simulink model "FOC_xeConCauTruc_discrete_251130_DNQ"  (R2024b)
settings: Solver=ode1  StartTime=0.0  StopTime=110  FixedStep=Tsample  MaxStep=1e-3  RelTol=1e-6  EnableMultiTasking=on
values from neighbouring files (symbols this model uses):
  ki1 = kp1/Ti1    (= 1470.9983644)    [parameters.m]    (also in thongso.m = 740.192826747)
  ki2 = kp2/Ti2    (= 348.309892151)    [parameters.m]    (also in thongso.m = 697.25500171)
  kp1 = Ti1/(k*5*(1/4000))    (= 14.8818990391)    [parameters.m]    (also in thongso.m = 10.2896717027)
  kp2 = 2*eta*0.0676/(KT*T0w)    (= 3.04771155633)    [parameters.m]    (also in thongso.m = 4.88078501197)
  Llr = 0.009662862    [parameters.m]    (also in thongso.m = 0.005238655)
  Lls = 0.009662862    [parameters.m]    (also in thongso.m = 0.005238655)
  Lm = 0.1213    [parameters.m]    (also in thongso.m = 0.141018834)
  p = 4    [parameters.m]    (also in thongso.m = 2)
  P = 8    [parameters.m]    (also in thongso.m = 4)
  Rr = 0.97664535    [parameters.m]    (also in thongso.m = 0.380952381)
  Rs = 1.000830856    [parameters.m]    (also in thongso.m = 0.386041637)
  Tr = Lr/Rr    (= 0.134088592138)    [parameters.m]    (also in thongso.m = 0.383925908577)
  Ts = Ls/Rs    (= 0.130848781505)    [parameters.m]    (also in thongso.m = 0.378864544604)
  Tsample = 1e-5    (= 1e-05)    [parameters.m]    (also in thongso.m)
  Vdc = 900    [parameters.m]    (also in thongso.m = 510)
undefined symbols (not defined in the file or in its folder): DiscIntNeverNeededParam, dspblkCoreblockFVToolHelper, gcbh
libraries: powerlib_extras x5, slpidlib x3, spsUniversalBridgeLib x1, spsAsynchronousMachineSIUnitsLib x1, simulink x1, spsVoltageMeasurementLib x1, spsDCVoltageSourceLib x1, sps_lib x1, SignalEditorBlockLib x1
settings Model: Creator=Dell  LastModifiedBy=Admin
settings SolverCC: AlgebraicLoopSolver=TrustRegion
settings DataIOCC: LimitDataPoints=on  SaveFormat=Array  SignalLoggingSaveFormat=ModelDataLogs  ReturnWorkspaceOutputs=off
settings OptimizationCC: ExpressionDepthLimit=2147483647  LifeSpan=inf
settings DebuggingCC: UnderspecifiedInitializationDetection=Classic  MergeDetectMultiDrivingBlocksExec=none  SolverPrmCheckMsg=warning  FcnCallInpInsideContextMsg=warning  UnconnectedInputMsg=warning  UnconnectedOutputMsg=warning  UnconnectedLineMsg=warning  StateNameClashWarn=warning  SFUnexpectedBacktrackingDiag=warning  SFNoUnconditionalDefaultTransitionDiag=warning  ArithmeticOperatorsInVariantConditions=warning
settings HardwareCC: ProdBitPerPointer=32  ProdBitPerSizeT=32  ProdBitPerPtrDiffT=32  ProdLargestAtomicFloat=None  ProdIntDivRoundTo=Undefined  ProdEndianess=Unspecified  ProdWordSize=32  ProdHWDeviceType=32-bit Generic
settings ModelReferenceCC: EnableRefExpFcnMdlSchedulingChecks=on  PropagateSignalLabelsOutOfModel=off
settings SFSimCC: SimUseLocalCustomCode=off  SimParseCustomCode=off  CustomCodeUndefinedFunction=UseInterfaceOnly
settings RTWCC: RTWUseLocalCustomCode=off  GPUComputeCapability=3.5
settings CodeAppCC: StateflowObjectComments=on
settings GRTTargetCC: TargetLangStandard=C89/C90 (ANSI)  CombineOutputUpdateFcns=off  GRTInterface=on
settings ConfigComp: CovMetricSettings=dw  CovSaveCumulativeToWorkspaceVar=on  CovSaveSingleToWorkspaceVar=on  CovExternalEMLEnable=off  CovSFcnEnable=off
settings SimscapeCC: SimscapeNormalizeSystem=off

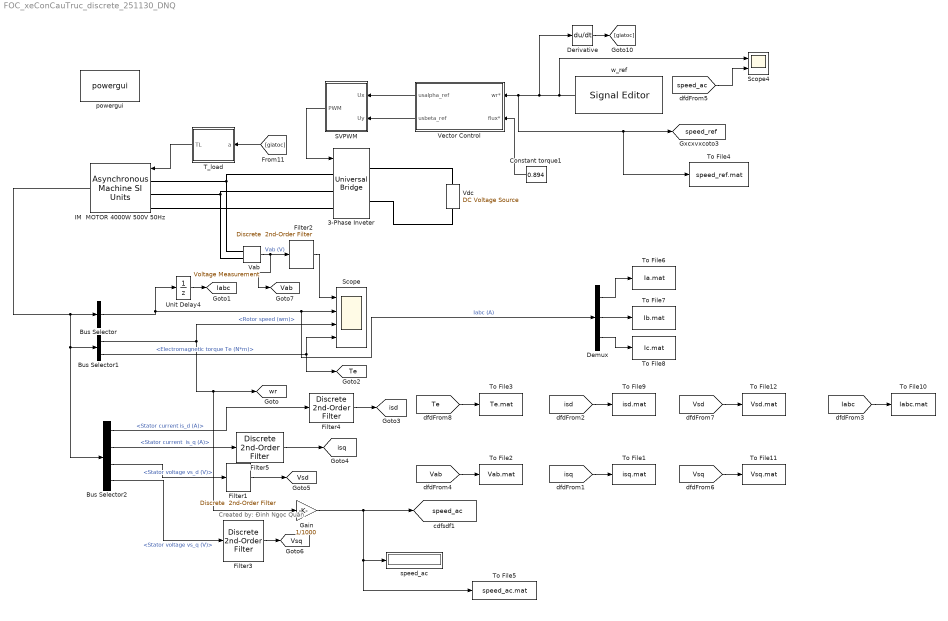
== system FOC_xeConCauTruc_discrete_251130_DNQ ==
  note: Created by: Đinh Ngọc Quân
  3-Phase Inveter : spsUniversalBridgeLib/Universal Bridge  Arms=3  SnubberResistance=1e5  SnubberCapacitance=1e-6  Device=IGBT / Diodes  Ron=1e-3  Lon=0  ForwardVoltages="[1.1  0.75]"  ForwardVoltage=0  GTOparameters=[ 10e-6 , 20e-6 ]  IGBTparameters=[ 1e-6 , 2e-6 ]  Measurements=None  Measurements_2=None  converterType=Rectifier
  Bus Selector : BusSelector  OutputSignals=Stator measurements.Stator current is_a (A),Stator measurements.Stator current is_b (A),Stator measurements.Stator current is_c (A)  OutputAsBus=on
  Bus Selector1 : BusSelector  OutputSignals=Mechanical.Rotor speed (wm),Mechanical.Electromagnetic torque Te (N*m)
  Bus Selector2 : BusSelector  OutputSignals="Stator measurements.Stator current is_d (A),Stator measurements.Stator current  is_q (A),Stator measurements.Stator voltage vs_d (V),Stator measurements.Stator voltage vs_q (V)"
  Constant torque1 : Constant  Value=0.894
  Demux : Demux  Outputs=3
  Derivative : Derivative
  Filter{1..5} (5 alike) : powerlib_extras/Discrete  Control Blocks/Discrete  2nd-Order Filter  FilterType=Lowpass  Fo=100  Zeta=0.707  Ts=Tsample  Initialize=off  Vac_Init=[0.8 -25 60]  Vdc_Init=-0.4  PlotResponse=off  param1=[1 500 1]
  Gain : Gain  Gain=1/1000
  IM  MOTOR 4000W 500V 50Hz : spsAsynchronousMachineSIUnitsLib/Asynchronous Machine SI Units  RotorType=Squirrel-cage  PresetModel=No  MechanicalLoad=Torque Tm  ShowDetailedParameters=on  ReferenceFrame=Rotor  Units=SI  MeasurementBus=off  NominalParameters=[4000 400 50]  VoltageRatio=1  Stator=[Rs Lls]  Rotor=[Rr Llr]  Cage1=[0.4155 0.002066]  Cage2=[0.4168 0.0003495]  Lm=Lm  Mechanical=[0.0676 0 p]  PolePairs=2  InitialConditions=[1 0 0 0 0 0 0 0]  SimulateSaturation=off  Saturation=[14.03593122, 27.81365428, 53.79336849, 72.68890987, 97.98006896, 148.6815601, 215.7428561, 302.9841135, 428.7778367 ; 230, 322, 414, 460, 506, 552, 598, 644, 690]  LoadFlowParameters=1492000  TsPowergui=0  TsBlock=-1  IterativeModel=Trapezoidal non iterative  IterativeDiscreteModel=Trapezoidal non iterative  Pmec=1.492e+006
  SVPWM : Subsystem
  Scope : Scope  NumInputPorts=4
  Scope4 : Scope  NumInputPorts=2
  T_load : Subsystem
  To File1 : ToFile  Filename=isq.mat  MatrixName=isq
  To File10 : ToFile  Filename=Iabc.mat  MatrixName=Iabc
  To File11 : ToFile  Filename=Vsq.mat  MatrixName=Vsq
  To File12 : ToFile  Filename=Vsd.mat  MatrixName=Vsd
  To File2 : ToFile  Filename=Vab.mat  MatrixName=Vab
  To File3 : ToFile  Filename=Te.mat  MatrixName=Te
  To File4 : ToFile  Filename=speed_ref.mat  MatrixName=speed_ref
  To File5 : ToFile  Filename=speed_ac.mat  MatrixName=speed_ac
  To File6 : ToFile  Filename=Ia.mat  MatrixName=Ia
  To File7 : ToFile  Filename=Ib.mat  MatrixName=Ib
  To File8 : ToFile  Filename=Ic.mat  MatrixName=Ic
  To File9 : ToFile  Filename=isd.mat  MatrixName=isd
  Unit Delay4 : UnitDelay  SampleTime=Tsample  HasFrameUpgradeWarning=on
  Vab : spsVoltageMeasurementLib/Voltage Measurement  Tag=PoWeRsYsTeMmEaSuReMeNt  PhasorSimulation=off  OutputType=Magnitude  PSBequivalent=0
  Vdc : spsDCVoltageSourceLib/DC Voltage Source  Amplitude=Vdc  Measurements=None
  Vector Control : Subsystem
  powergui : sps_lib/powergui  Priority=2  SimulationMode=Discrete  SampleTime=Tsample  frequency=60  Iterations=50  frequencyindice=50  Pbase=100e6  ErrMax=1e-4  UnitsV=kV  UnitsW=MW  buscounter=0  FunctionMessages=off  echomessages=off  EnableUseOfTLC=off  CurrentSourceSwitches=off  DisableSnubberDevices=off  DisableRonSwitches=off  DisableVfSwitches=off  DisplayEquations=off  AutomaticDiscreteSolvers=off  SolverType=Tustin/Backward Euler (TBE)  Interpol=off  ExternalGateDelay=off  methode=off  Ts=0  x0status=blocks  SPID=off  SwTol=0  HookPort=off  NonlinearTolerance=0  nMaxIteration=15  ContinueOnMaxIteration=off  RestoreLinks=warning  ResistiveCurrentMeasurement=off  Frange=[0:2:500]  Ylog=off  Xlog=on  ShowGrid=off  save=off  variable=ZData  structure=0  ZoomFFT=on  StartTime=0.0  cycles=1  DisplayStyle=off  fundamental=60  FreqAxis=off  MaxFrequency=1000  frequencyindicesteady=1  RmsSteady=1  display=off
  speed_ac : Display
  w_ref : SignalEditorBlockLib/Signal Editor  FileName=velocity_ref.mat  ActiveScenario=Scenario  ActiveSignal=Signal 1  IsBus=off  OutputBusObjectStr=Bus: BusObject  SampleTime=0  ZeroCross=off  OutputAfterFinalValue=Setting to zero  Unit=inherit  PreserveSignalName=on  ApplySigPropsToAllScenarios=on  ApplySigPropsToAllSignals=off
  tag scope: Iabc=global, Te=global, Vab=global, Vsd=global, Vsq=global, isd=global, isq=global, speed_ac=global, speed_ref=global, wr=global
  wires:
  Bus Selector1/1 -> Scope/3, Gain/1, [wr]  "<Rotor speed (wm)>"
  Bus Selector/1 -> Unit Delay4/1, Demux/1, Scope/2  "Iabc (A)"
  Bus Selector1/2 -> Scope/4, [Te]  "<Electromagnetic torque Te (N*m)>"
  IM  MOTOR 4000W 500V 50Hz/1 -> Bus Selector2/1, Bus Selector1/1, Bus Selector/1
  Constant torque1/1 -> Vector Control/2(flux*)
  Vector Control/1(usalpha_ref) -> SVPWM/1(Ux)
  Vector Control/2(usbeta_ref) -> SVPWM/2(Uy)
  SVPWM/1(PWM) -> 3-Phase Inveter/1
  Vab/1 -> [Vab], Filter2/1  "Vab (V)"
  Filter2/1 -> Scope/1
  Bus Selector2/3 -> Filter1/1  "<Stator voltage vs_d (V)>"
  Filter1/1 -> [Vsd]
  Bus Selector2/4 -> Filter3/1  "<Stator voltage vs_q (V)>"
  Filter3/1 -> [Vsq]
  Bus Selector2/1 -> Filter4/1  "<Stator current is_d (A)>"
  Bus Selector2/2 -> Filter5/1  "<Stator current  is_q (A)>"
  Filter4/1 -> [isd]
  Filter5/1 -> [isq]
  [Te] -> To File3/1
  [Vab] -> To File2/1
  Demux/1 -> To File6/1
  Demux/3 -> To File8/1
  Demux/2 -> To File7/1
  Unit Delay4/1 -> [Iabc]
  [isq] -> To File1/1
  [isd] -> To File9/1
  [Vsq] -> To File11/1
  [Vsd] -> To File12/1
  [Iabc] -> To File10/1
  T_load/1(TL) -> IM  MOTOR 4000W 500V 50Hz/1
  w_ref/1 -> Scope4/1, Derivative/1, Vector Control/1(wr*), To File4/1, [speed_ref]
  Derivative/1 -> [giatoc]
  [giatoc] -> T_load/1(a)
  [speed_ac] -> Scope4/2
  Gain/1 -> [speed_ac], speed_ac/1, To File5/1
  connections:
  IM  MOTOR 4000W 500V 50Hz/LConn2 -- 3-Phase Inveter/LConn2 -- Vab/LConn2
  IM  MOTOR 4000W 500V 50Hz/LConn1 -- 3-Phase Inveter/LConn1 -- Vab/LConn1
  IM  MOTOR 4000W 500V 50Hz/LConn3 -- 3-Phase Inveter/LConn3
  3-Phase Inveter/RConn1 -- Vdc/RConn1
  Vdc/LConn1 -- 3-Phase Inveter/RConn2

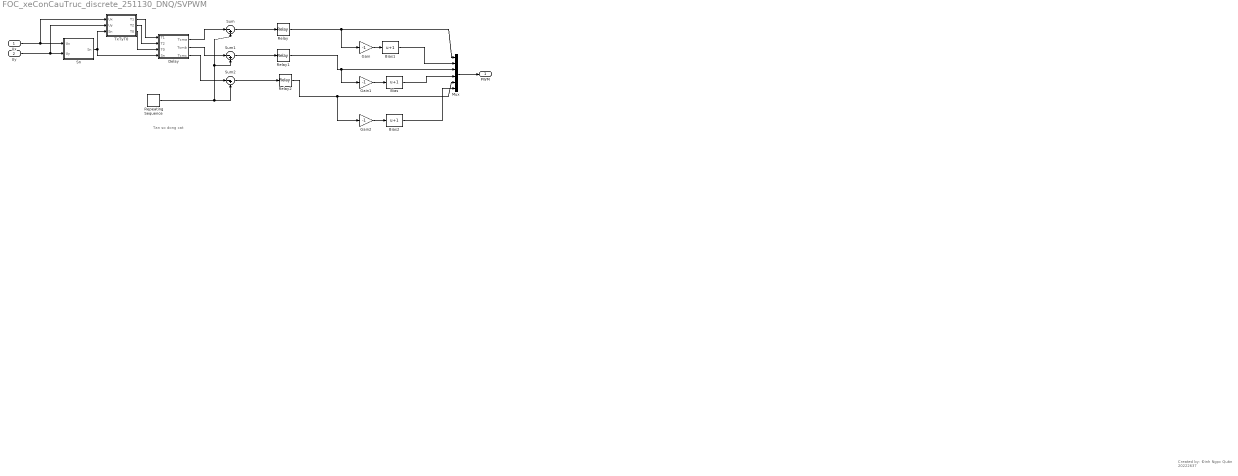
== system FOC_xeConCauTruc_discrete_251130_DNQ/SVPWM ==
  note: Tan so dong cat
  note: Created by: Đinh Ngọc Quân 20222637
  Ux : Inport
  Uy : Inport  Port=2
  Bias : Bias  Bias=1  SaturateOnIntegerOverflow=off
  Bias1 : Bias  Bias=1  SaturateOnIntegerOverflow=off
  Bias2 : Bias  Bias=1  SaturateOnIntegerOverflow=off
  Delay : MATLAB Function  TreatAsAtomicUnit=on
  Gain : Gain  Gain=-1
  Gain1 : Gain  Gain=-1
  Gain2 : Gain  Gain=-1
  Mux : Mux  Inputs=6
  Relay : Relay  OnSwitchValue=0  OffSwitchValue=0
  Relay1 : Relay  OnSwitchValue=0  OffSwitchValue=0
  Relay2 : Relay  OnSwitchValue=0  OffSwitchValue=0
  Repeating Sequence : simulink/Sources/Repeating Sequence  rep_seq_t=[0 1/5000/2 1/5000]  rep_seq_y=[0 1/2000/2 0]
  Sn : MATLAB Function  TreatAsAtomicUnit=on
  Sum : Sum  Inputs=|-+
  Sum1 : Sum  Inputs=|-+
  Sum2 : Sum  Inputs=|-+
  TxTyT0 : MATLAB Function  TreatAsAtomicUnit=on
  PWM : Outport  VectorParamsAs1DForOutWhenUnconnected=off
  wires:
  Delay/1(Tcma) -> Sum/1
  Delay/2(Tcmb) -> Sum1/1
  Delay/3(Tcmc) -> Sum2/1
  Repeating Sequence/1 -> Sum/2, Sum1/2, Sum2/2
  Sum/1 -> Relay/1
  Sum2/1 -> Relay2/1
  Sum1/1 -> Relay1/1
  Relay1/1 -> Mux/3, Gain1/1
  Relay2/1 -> Mux/5, Gain2/1
  Sn/1(Sn) -> TxTyT0/3(Sn), Delay/4(Sn)
  TxTyT0/1(T1) -> Delay/1(T1)
  TxTyT0/2(T2) -> Delay/2(T2)
  TxTyT0/3(T0) -> Delay/3(T0)
  Mux/1 -> PWM/1
  Gain1/1 -> Bias/1
  Gain/1 -> Bias1/1
  Gain2/1 -> Bias2/1
  Bias1/1 -> Mux/2
  Bias/1 -> Mux/4
  Bias2/1 -> Mux/6
  Relay/1 -> Mux/1, Gain/1
  Ux/1 -> Sn/1(Ux), TxTyT0/1(Ux)
  Uy/1 -> Sn/2(Uy), TxTyT0/2(Uy)

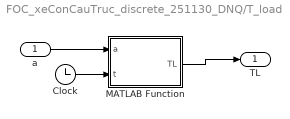
== system FOC_xeConCauTruc_discrete_251130_DNQ/T_load ==
  a : Inport
  Clock : Clock
  MATLAB Function : MATLAB Function  TreatAsAtomicUnit=on
  TL : Outport
  wires:
  a/1 -> MATLAB Function/1(a)
  MATLAB Function/1(TL) -> TL/1
  Clock/1 -> MATLAB Function/2(t)

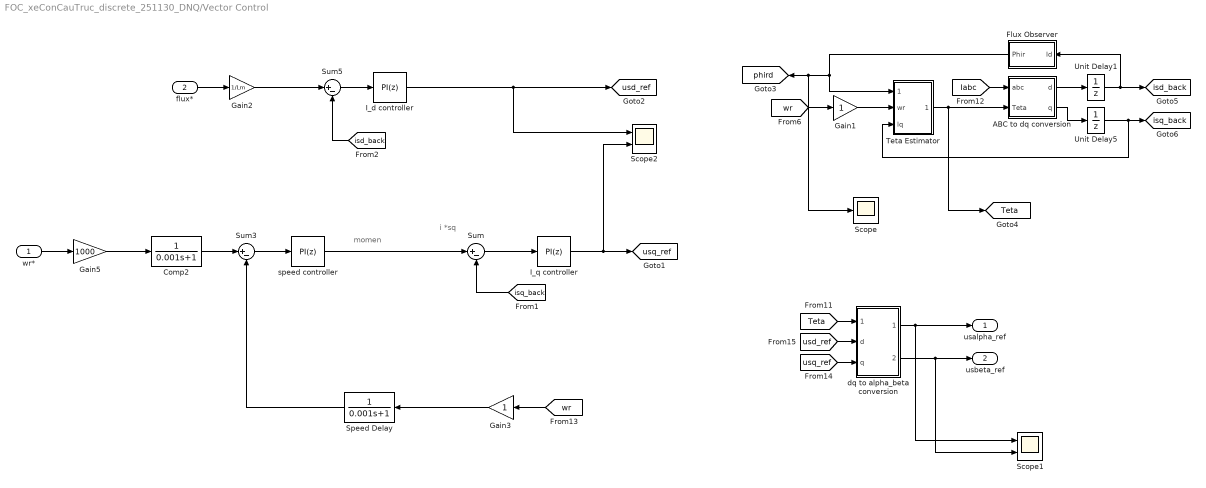
== system FOC_xeConCauTruc_discrete_251130_DNQ/Vector Control ==
  note: momen
  note: i *sq
  wr* : Inport
  flux* : Inport  Port=2
  ABC to dq conversion : Subsystem
  Comp2 : TransferFcn  Denominator=[0.001 1]
  Flux Observer : Subsystem
  Gain1 : Gain
  Gain2 : Gain  Gain=1/Lm
  Gain3 : Gain
  Gain5 : Gain  Gain=1000
  I_d controller : slpidlib/PID Controller  Controller=PI  Form=Parallel  TimeDomain=Discrete-time  UseExternalTs=off  SampleTime=-1  IntegratorMethod=Forward Euler  FilterMethod=Forward Euler  ControllerParametersSource=internal  P=kp1  I=ki1  UseKiTs=off  D=0  UseExternalDerivativeSource=off  N=100  UseFilter=on  TunerSelectOption=Transfer Function Based (PID Tuner App)  InitialConditionSource=internal  InitialConditionForIntegrator=0  InitialConditionForFilter=0  DifferentiatorICPrevScaledInput=0  ExternalReset=none  TrackingMode=off  Kt=1  LimitOutput=off  SatLimitsSource=internal  UpperSaturationLimit=inf  LowerSaturationLimit=-inf  LinearizeAsGain=on  AntiWindupMode=none  Kb=1  LimitIntegrator=off  UpperIntegratorSaturationLimit=inf  LowerIntegratorSaturationLimit=-inf  POutMin=[]  POutMax=[]  IOutMin=[]  IOutMax=[]  DOutMin=[]  DOutMax=[]  NOutMin=[]  NOutMax=[]  SumOutMin=[]  SumOutMax=[]  SaturationOutMin=[]  SaturationOutMax=[]  PParamMin=[]  PParamMax=[]  IParamMin=[]  IParamMax=[]  DParamMin=[]  DParamMax=[]  NParamMin=[]  NParamMax=[]  KbParamMin=[]  KbParamMax=[]  KtParamMin=[]  KtParamMax=[]  KbOutMin=[]  KbOutMax=[]  KtOutMin=[]  KtOutMax=[]  IntegratorOutMin=[]  IntegratorOutMax=[]  FilterOutMin=[]  FilterOutMax=[]  SumI1OutMin=[]  SumI1OutMax=[]  SumI2OutMin=[]  SumI2OutMax=[]  SumI3OutMin=[]  SumI3OutMax=[]  SumI4OutMin=[]  SumI4OutMax=[]  SumDOutMin=[]  SumDOutMax=[]  DifferentiatorOutMin=[]  DifferentiatorOutMax=[]  FilterDiffOutCoefMin=[]  FilterDiffOutCoefMax=[]  ReciprocalOutMin=[]  ReciprocalOutMax=[]  SumDenOutMin=[]  SumDenOutMax=[]  SumNumOutMin=[]  SumNumOutMax=[]  DivideOutMin=[]  DivideOutMax=[]  UdiffTsProdOutMin=[]  UdiffTsProdOutMax=[]  NTsProdOutMin=[]  NTsProdOutMax=[]  UintegralTsProdOutMin=[]  UintegralTsProdOutMax=[]  UngainTsProdOutMin=[]  UngainTsProdOutMax=[]  ClampingZeroOutDataTypeStr=Inherit: Inherit via back propagation  ClampingZeroOutMin=[]  ClampingZeroOutMax=[]  FilterDenConstantOutDataTypeStr=Inherit: Inherit via back propagation  FilterDenConstantOutMin=[]  FilterDenConstantOutMax=[]  PCopyOutDataTypeStr=Inherit: Inherit via back propagation  PCopyOutMin=[]  PCopyOutMax=[]  NCopyOutDataTypeStr=Inherit: Inherit via back propagation  NCopyOutMin=[]  NCopyOutMax=[]  IntegratorContinuousStateAttributes=''  IntegratorStateMustResolveToSignalObject=off  IntegratorRTWStateStorageClass=Auto  FilterContinuousStateAttributes=''  FilterStateMustResolveToSignalObject=off  FilterRTWStateStorageClass=Auto  ParallelPVariant=InternalParameters  IdealPVariant=Disabled  IVariant=InternalParameters  DVariant=Disabled  IntegratorVariant=Discrete  SatVariant=Disabled  AWVariant=Passthrough  PCopyVariant=Disabled  TRVariant=Disabled  FdbkBlocksVariant=Forward  IdealPFdbkVariant=Disabled  SatFdbkVariant=Disabled  DerivativeFilterVariant=Disabled  NVariant=Disabled  NCopyVariant=Disabled_SignalSpec  FilterICVariant=Disabled  IntegratorICVariant=InternalICs  ExternalResetVariant=Disabled  TRSumVariant=Passthrough  SumFdbkVariant=Disabled  SumVariant=Sum_PI  TsampFilterVariant=InternalTs  TsampNgainVariant=Passthrough  TsampIntegralVariant=Disabled_SignalSpec  ExternalSaturationOutDataTypeStr=Inherit: Same as second input  DerivativeSourceVariant=Disabled  PreIntVariant=InternalPreInt
  I_q controller : slpidlib/PID Controller  Controller=PI  Form=Parallel  TimeDomain=Discrete-time  UseExternalTs=off  SampleTime=-1  IntegratorMethod=Forward Euler  FilterMethod=Forward Euler  ControllerParametersSource=internal  P=kp1  I=ki1  UseKiTs=off  D=0  UseExternalDerivativeSource=off  N=100  UseFilter=on  TunerSelectOption=Transfer Function Based (PID Tuner App)  InitialConditionSource=internal  InitialConditionForIntegrator=0  InitialConditionForFilter=0  DifferentiatorICPrevScaledInput=0  ExternalReset=none  TrackingMode=off  Kt=1  LimitOutput=off  SatLimitsSource=internal  UpperSaturationLimit=inf  LowerSaturationLimit=-inf  LinearizeAsGain=on  AntiWindupMode=none  Kb=1  LimitIntegrator=off  UpperIntegratorSaturationLimit=inf  LowerIntegratorSaturationLimit=-inf  POutMin=[]  POutMax=[]  IOutMin=[]  IOutMax=[]  DOutMin=[]  DOutMax=[]  NOutMin=[]  NOutMax=[]  SumOutMin=[]  SumOutMax=[]  SaturationOutMin=[]  SaturationOutMax=[]  PParamMin=[]  PParamMax=[]  IParamMin=[]  IParamMax=[]  DParamMin=[]  DParamMax=[]  NParamMin=[]  NParamMax=[]  KbParamMin=[]  KbParamMax=[]  KtParamMin=[]  KtParamMax=[]  KbOutMin=[]  KbOutMax=[]  KtOutMin=[]  KtOutMax=[]  IntegratorOutMin=[]  IntegratorOutMax=[]  FilterOutMin=[]  FilterOutMax=[]  SumI1OutMin=[]  SumI1OutMax=[]  SumI2OutMin=[]  SumI2OutMax=[]  SumI3OutMin=[]  SumI3OutMax=[]  SumI4OutMin=[]  SumI4OutMax=[]  SumDOutMin=[]  SumDOutMax=[]  DifferentiatorOutMin=[]  DifferentiatorOutMax=[]  FilterDiffOutCoefMin=[]  FilterDiffOutCoefMax=[]  ReciprocalOutMin=[]  ReciprocalOutMax=[]  SumDenOutMin=[]  SumDenOutMax=[]  SumNumOutMin=[]  SumNumOutMax=[]  DivideOutMin=[]  DivideOutMax=[]  UdiffTsProdOutMin=[]  UdiffTsProdOutMax=[]  NTsProdOutMin=[]  NTsProdOutMax=[]  UintegralTsProdOutMin=[]  UintegralTsProdOutMax=[]  UngainTsProdOutMin=[]  UngainTsProdOutMax=[]  ClampingZeroOutDataTypeStr=Inherit: Inherit via back propagation  ClampingZeroOutMin=[]  ClampingZeroOutMax=[]  FilterDenConstantOutDataTypeStr=Inherit: Inherit via back propagation  FilterDenConstantOutMin=[]  FilterDenConstantOutMax=[]  PCopyOutDataTypeStr=Inherit: Inherit via back propagation  PCopyOutMin=[]  PCopyOutMax=[]  NCopyOutDataTypeStr=Inherit: Inherit via back propagation  NCopyOutMin=[]  NCopyOutMax=[]  IntegratorContinuousStateAttributes=''  IntegratorStateMustResolveToSignalObject=off  IntegratorRTWStateStorageClass=Auto  FilterContinuousStateAttributes=''  FilterStateMustResolveToSignalObject=off  FilterRTWStateStorageClass=Auto  ParallelPVariant=InternalParameters  IdealPVariant=Disabled  IVariant=InternalParameters  DVariant=Disabled  IntegratorVariant=Discrete  SatVariant=Disabled  AWVariant=Passthrough  PCopyVariant=Disabled  TRVariant=Disabled  FdbkBlocksVariant=Forward  IdealPFdbkVariant=Disabled  SatFdbkVariant=Disabled  DerivativeFilterVariant=Disabled  NVariant=Disabled  NCopyVariant=Disabled_SignalSpec  FilterICVariant=Disabled  IntegratorICVariant=InternalICs  ExternalResetVariant=Disabled  TRSumVariant=Passthrough  SumFdbkVariant=Disabled  SumVariant=Sum_PI  TsampFilterVariant=InternalTs  TsampNgainVariant=Passthrough  TsampIntegralVariant=Disabled_SignalSpec  ExternalSaturationOutDataTypeStr=Inherit: Same as second input  DerivativeSourceVariant=Disabled  PreIntVariant=InternalPreInt
  Scope : Scope
  Scope1 : Scope  NumInputPorts=2
  Scope2 : Scope  NumInputPorts=2
  Speed Delay : TransferFcn  Denominator=[0.001 1]
  Sum : Sum  Inputs=|+-
  Sum3 : Sum  Inputs=|+-
  Sum5 : Sum  Inputs=|+-
  Teta Estimator : Subsystem
  Unit Delay1 : UnitDelay  SampleTime=Tsample  HasFrameUpgradeWarning=on
  Unit Delay5 : UnitDelay  SampleTime=Tsample  HasFrameUpgradeWarning=on
  dq to alpha_beta conversion : Subsystem
  speed controller : slpidlib/PID Controller  Controller=PI  Form=Parallel  TimeDomain=Discrete-time  UseExternalTs=off  SampleTime=-1  IntegratorMethod=Forward Euler  FilterMethod=Forward Euler  ControllerParametersSource=internal  P=kp2  I=ki2  UseKiTs=off  D=0  UseExternalDerivativeSource=off  N=100  UseFilter=on  TunerSelectOption=Transfer Function Based (PID Tuner App)  InitialConditionSource=internal  InitialConditionForIntegrator=0  InitialConditionForFilter=0  DifferentiatorICPrevScaledInput=0  ExternalReset=none  TrackingMode=off  Kt=1  LimitOutput=off  SatLimitsSource=internal  UpperSaturationLimit=inf  LowerSaturationLimit=-inf  LinearizeAsGain=on  AntiWindupMode=none  Kb=1  LimitIntegrator=off  UpperIntegratorSaturationLimit=inf  LowerIntegratorSaturationLimit=-inf  POutMin=[]  POutMax=[]  IOutMin=[]  IOutMax=[]  DOutMin=[]  DOutMax=[]  NOutMin=[]  NOutMax=[]  SumOutMin=[]  SumOutMax=[]  SaturationOutMin=[]  SaturationOutMax=[]  PParamMin=[]  PParamMax=[]  IParamMin=[]  IParamMax=[]  DParamMin=[]  DParamMax=[]  NParamMin=[]  NParamMax=[]  KbParamMin=[]  KbParamMax=[]  KtParamMin=[]  KtParamMax=[]  KbOutMin=[]  KbOutMax=[]  KtOutMin=[]  KtOutMax=[]  IntegratorOutMin=[]  IntegratorOutMax=[]  FilterOutMin=[]  FilterOutMax=[]  SumI1OutMin=[]  SumI1OutMax=[]  SumI2OutMin=[]  SumI2OutMax=[]  SumI3OutMin=[]  SumI3OutMax=[]  SumI4OutMin=[]  SumI4OutMax=[]  SumDOutMin=[]  SumDOutMax=[]  DifferentiatorOutMin=[]  DifferentiatorOutMax=[]  FilterDiffOutCoefMin=[]  FilterDiffOutCoefMax=[]  ReciprocalOutMin=[]  ReciprocalOutMax=[]  SumDenOutMin=[]  SumDenOutMax=[]  SumNumOutMin=[]  SumNumOutMax=[]  DivideOutMin=[]  DivideOutMax=[]  UdiffTsProdOutMin=[]  UdiffTsProdOutMax=[]  NTsProdOutMin=[]  NTsProdOutMax=[]  UintegralTsProdOutMin=[]  UintegralTsProdOutMax=[]  UngainTsProdOutMin=[]  UngainTsProdOutMax=[]  ClampingZeroOutDataTypeStr=Inherit: Inherit via back propagation  ClampingZeroOutMin=[]  ClampingZeroOutMax=[]  FilterDenConstantOutDataTypeStr=Inherit: Inherit via back propagation  FilterDenConstantOutMin=[]  FilterDenConstantOutMax=[]  PCopyOutDataTypeStr=Inherit: Inherit via back propagation  PCopyOutMin=[]  PCopyOutMax=[]  NCopyOutDataTypeStr=Inherit: Inherit via back propagation  NCopyOutMin=[]  NCopyOutMax=[]  IntegratorContinuousStateAttributes=''  IntegratorStateMustResolveToSignalObject=off  IntegratorRTWStateStorageClass=Auto  FilterContinuousStateAttributes=''  FilterStateMustResolveToSignalObject=off  FilterRTWStateStorageClass=Auto  ParallelPVariant=InternalParameters  IdealPVariant=Disabled  IVariant=InternalParameters  DVariant=Disabled  IntegratorVariant=Discrete  SatVariant=Disabled  AWVariant=Passthrough  PCopyVariant=Disabled  TRVariant=Disabled  FdbkBlocksVariant=Forward  IdealPFdbkVariant=Disabled  SatFdbkVariant=Disabled  DerivativeFilterVariant=Disabled  NVariant=Disabled  NCopyVariant=Disabled_SignalSpec  FilterICVariant=Disabled  IntegratorICVariant=InternalICs  ExternalResetVariant=Disabled  TRSumVariant=Passthrough  SumFdbkVariant=Disabled  SumVariant=Sum_PI  TsampFilterVariant=InternalTs  TsampNgainVariant=Passthrough  TsampIntegralVariant=Disabled_SignalSpec  ExternalSaturationOutDataTypeStr=Inherit: Same as second input  DerivativeSourceVariant=Disabled  PreIntVariant=InternalPreInt
  usalpha_ref : Outport  VectorParamsAs1DForOutWhenUnconnected=off
  usbeta_ref : Outport  Port=2  VectorParamsAs1DForOutWhenUnconnected=off
  tag scope: Teta=global, isd_back=global, isq_back=global, phird=global, usd_ref=global, usq_ref=global
  wires:
  Sum/1 -> I_q controller/1
  speed controller/1 -> Sum/1
  I_q controller/1 -> [usq_ref], Scope2/2
  [wr] -> Gain3/1
  Sum3/1 -> speed controller/1
  Gain5/1 -> Comp2/1
  Sum5/1 -> I_d controller/1
  Flux Observer/1(Phir) -> Teta Estimator/1(Phird), [phird], Scope/1
  Teta Estimator/1(Teta) -> ABC to dq conversion/2(Teta), [Teta]
  [wr] -> Gain1/1
  [Iabc] -> ABC to dq conversion/1(abc)
  [Teta] -> dq to alpha_beta conversion/1(Teta)
  wr*/1 -> Gain5/1
  ABC to dq conversion/1(d) -> Unit Delay1/1
  Unit Delay1/1 -> [isd_back], Flux Observer/1(Id)
  ABC to dq conversion/2(q) -> Unit Delay5/1
  Unit Delay5/1 -> Teta Estimator/3(Iq), [isq_back]
  [usd_ref] -> dq to alpha_beta conversion/2(d)
  [usq_ref] -> dq to alpha_beta conversion/3(q)
  Gain3/1 -> Speed Delay/1
  dq to alpha_beta conversion/1(usalpha) -> usalpha_ref/1, Scope1/1
  dq to alpha_beta conversion/2(usbeta) -> usbeta_ref/1, Scope1/2
  Gain1/1 -> Teta Estimator/2(wr)
  [isd_back] -> Sum5/2
  I_d controller/1 -> [usd_ref], Scope2/1
  [isq_back] -> Sum/2
  flux*/1 -> Gain2/1
  Gain2/1 -> Sum5/1
  Comp2/1 -> Sum3/1
  Speed Delay/1 -> Sum3/2

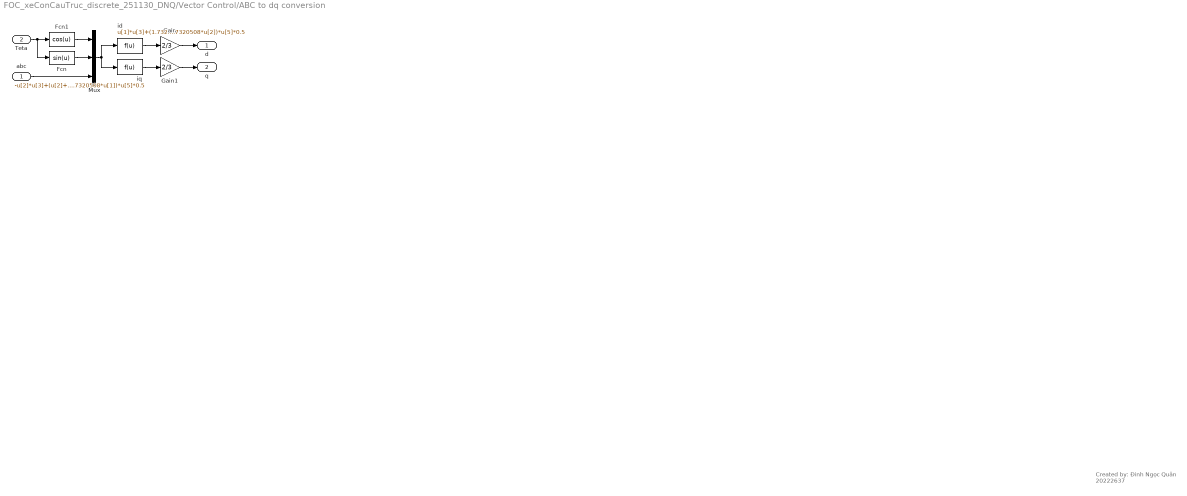
== system FOC_xeConCauTruc_discrete_251130_DNQ/Vector Control/ABC to dq conversion ==
  note: Created by: Đinh Ngọc Quân 20222637
  abc : Inport
  Teta : Inport  Port=2
  Fcn : Fcn  Expr=sin(u)
  Fcn1 : Fcn  Expr=cos(u)
  Gain : Gain  Gain=2/3  SaturateOnIntegerOverflow=on  OutDataTypeStr=Inherit: Same as input  ParamDataTypeStr=Inherit: Same as input
  Gain1 : Gain  Gain=2/3  SaturateOnIntegerOverflow=on  OutDataTypeStr=Inherit: Same as input  ParamDataTypeStr=Inherit: Same as input
  Mux : Mux  Inputs=[1 1 3]
  id : Fcn  Expr=u[1]*u[3]+(1.7320508*u[2]-u[1])*u[4]*0.5+(-u[1]-1.7320508*u[2])*u[5]*0.5
  iq : Fcn  Expr=-u[2]*u[3]+(u[2]+1.7320508*u[1])*u[4]*0.5+(u[2]-1.7320508*u[1])*u[5]*0.5
  d : Outport  InitialOutput=0  VectorParamsAs1DForOutWhenUnconnected=off
  q : Outport  Port=2  InitialOutput=0  VectorParamsAs1DForOutWhenUnconnected=off
  wires:
  Fcn/1 -> Mux/2
  Fcn1/1 -> Mux/1
  Teta/1 -> Fcn1/1, Fcn/1
  Mux/1 -> iq/1, id/1
  abc/1 -> Mux/3
  iq/1 -> Gain1/1
  id/1 -> Gain/1
  Gain/1 -> d/1
  Gain1/1 -> q/1

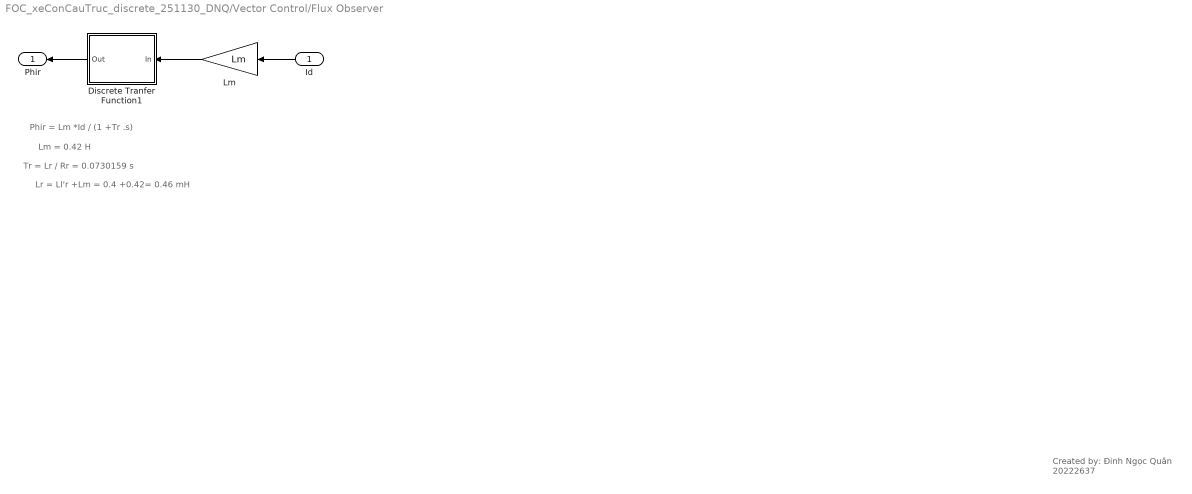
== system FOC_xeConCauTruc_discrete_251130_DNQ/Vector Control/Flux Observer ==
  note: Phir = Lm *Id / (1 +Tr .s)
  note: Lm = 0.42 H
  note: Lr = Ll'r +Lm = 0.4 +0.42= 0.46 mH
  note: Tr = Lr / Rr = 0.0730159 s
  note: Created by: Đinh Ngọc Quân 20222637
  Id : Inport
  Discrete Tranfer Function1 : Subsystem  mask(First Order Low Pass Filter (Discrete)){T=Tr, Ts=Ts}
      mask prompts: T "Time constant T (s) :"; Ts "Time step (s)"
      mask help: H(s)=1/(1+T.s)
      mask init:
      | X=[0 1 2 3 4];
      |  Y=[-2 -2 -3 -4 -4];
      |  str=sprintf('\nH=1/(1+T.s)\n T= %g s\n\n\n',T);
      | num=1;
      | den=[T 1];
      | 
      | % discrete transfer function
      | % descending powers of z
      | numd= Ts/T;
      | dend=[ 1  (Ts-T)/T];
      mask Display:
      | plot(X,Y);
      | disp(str);
  Lm : Gain  Gain=Lm  SaturateOnIntegerOverflow=on  OutDataTypeStr=Inherit: Same as input  ParamDataTypeStr=Inherit: Same as input
  Phir : Outport  VectorParamsAs1DForOutWhenUnconnected=off
  wires:
  Discrete Tranfer Function1/1(Out) -> Phir/1
  Id/1 -> Lm/1
  Lm/1 -> Discrete Tranfer Function1/1(In)

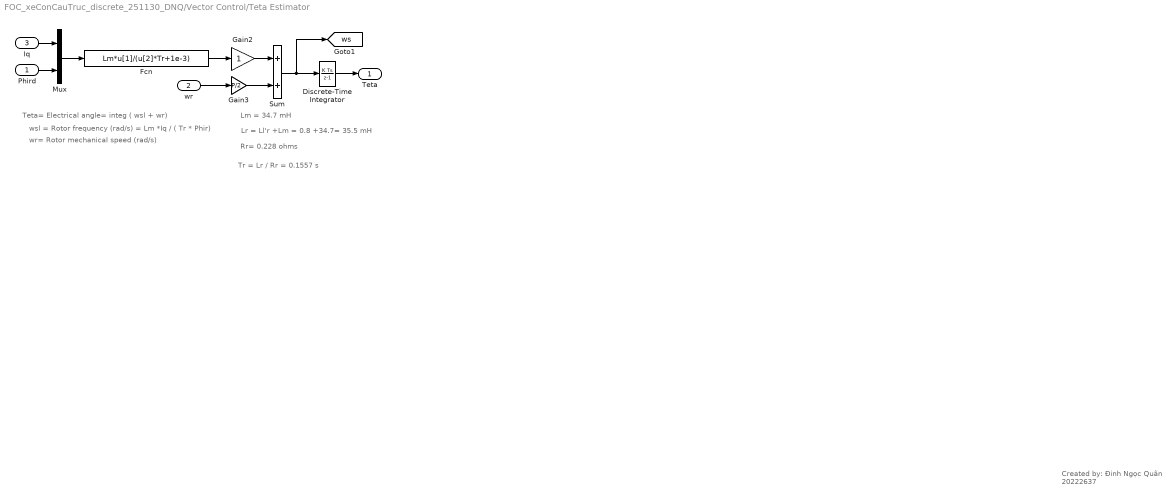
== system FOC_xeConCauTruc_discrete_251130_DNQ/Vector Control/Teta Estimator ==
  note: Teta= Electrical angle= integ ( wsl + wr)
  note: wsl = Rotor frequency (rad/s) = Lm *Iq / ( Tr * Phir)
  note: Lm = 34.7 mH
  note: Rr= 0.228 ohms
  note: Lr = Ll'r +Lm = 0.8 +34.7= 35.5 mH
  note: wr= Rotor mechanical speed (rad/s)
  note: Tr = Lr / Rr = 0.1557 s
  note: Created by: Đinh Ngọc Quân 20222637
  Phird : Inport
  wr : Inport  Port=2
  Iq : Inport  Port=3
  Discrete-Time Integrator : DiscreteIntegrator  SampleTime=Tsample  ICPrevOutput=DiscIntNeverNeededParam  ICPrevScaledInput=DiscIntNeverNeededParam
  Fcn : Fcn  Expr=Lm*u[1]/(u[2]*Tr+1e-3)
  Gain2 : Gain  SaturateOnIntegerOverflow=on  OutDataTypeStr=Inherit: Same as input  ParamDataTypeStr=Inherit: Same as input
  Gain3 : Gain  Gain=P/2  SaturateOnIntegerOverflow=on  OutDataTypeStr=Inherit: Same as input  ParamDataTypeStr=Inherit: Same as input
  Mux : Mux  Inputs=2
  Sum : Sum  InputSameDT=on  SaturateOnIntegerOverflow=on  OutDataTypeStr=Inherit: Same as first input
  Teta : Outport  InitialOutput=0  VectorParamsAs1DForOutWhenUnconnected=off
  tag scope: ws=global
  wires:
  Discrete-Time Integrator/1 -> Teta/1
  Sum/1 -> Discrete-Time Integrator/1, [ws]
  Gain3/1 -> Sum/2
  Gain2/1 -> Sum/1
  wr/1 -> Gain3/1
  Fcn/1 -> Gain2/1
  Phird/1 -> Mux/2
  Iq/1 -> Mux/1
  Mux/1 -> Fcn/1

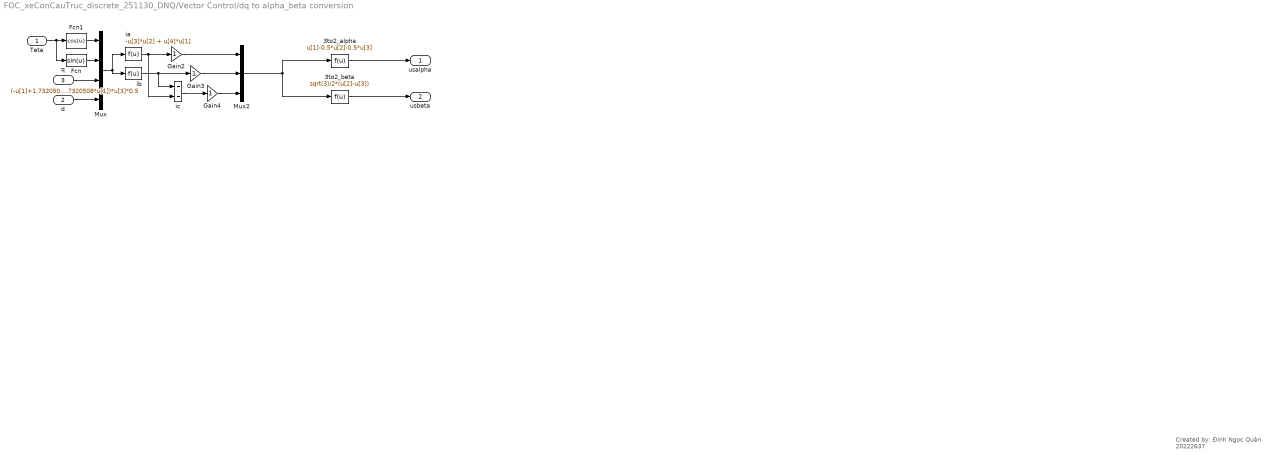
== system FOC_xeConCauTruc_discrete_251130_DNQ/Vector Control/dq to alpha_beta conversion ==
  note: Created by: Đinh Ngọc Quân 20222637
  Teta : Inport
  d : Inport  Port=2
  q : Inport  Port=3
  3to2_alpha : Fcn  Expr=u[1]-0.5*u[2]-0.5*u[3]
  3to2_beta : Fcn  Expr=sqrt(3)/2*(u[2]-u[3])
  Fcn : Fcn  Expr=sin(u)
  Fcn1 : Fcn  Expr=cos(u)
  Gain2 : Gain  SaturateOnIntegerOverflow=on  OutDataTypeStr=Inherit: Same as input  ParamDataTypeStr=Inherit: Same as input
  Gain3 : Gain  SaturateOnIntegerOverflow=on  OutDataTypeStr=Inherit: Same as input  ParamDataTypeStr=Inherit: Same as input
  Gain4 : Gain  SaturateOnIntegerOverflow=on  OutDataTypeStr=Inherit: Same as input  ParamDataTypeStr=Inherit: Same as input
  Mux : Mux
  Mux2 : Mux  Inputs=3
  ia : Fcn  Expr=-u[3]*u[2] + u[4]*u[1]
  ib : Fcn  Expr=(-u[1]+1.7320508*u[2])*u[4]*0.5+(u[2]+1.7320508*u[1])*u[3]*0.5
  ic : Sum  Inputs=--  InputSameDT=on  SaturateOnIntegerOverflow=on  OutDataTypeStr=Inherit: Same as first input
  usalpha : Outport  VectorParamsAs1DForOutWhenUnconnected=off
  usbeta : Outport  Port=2  VectorParamsAs1DForOutWhenUnconnected=off
  wires:
  Fcn/1 -> Mux/2
  Fcn1/1 -> Mux/1
  Mux/1 -> ib/1, ia/1
  Teta/1 -> Fcn1/1, Fcn/1
  q/1 -> Mux/3
  d/1 -> Mux/4
  Gain3/1 -> Mux2/2
  ic/1 -> Gain4/1
  Gain4/1 -> Mux2/3
  Gain2/1 -> Mux2/1
  ia/1 -> Gain2/1, ic/2
  ib/1 -> Gain3/1, ic/1
  Mux2/1 -> 3to2_alpha/1, 3to2_beta/1
  3to2_alpha/1 -> usalpha/1
  3to2_beta/1 -> usbeta/1

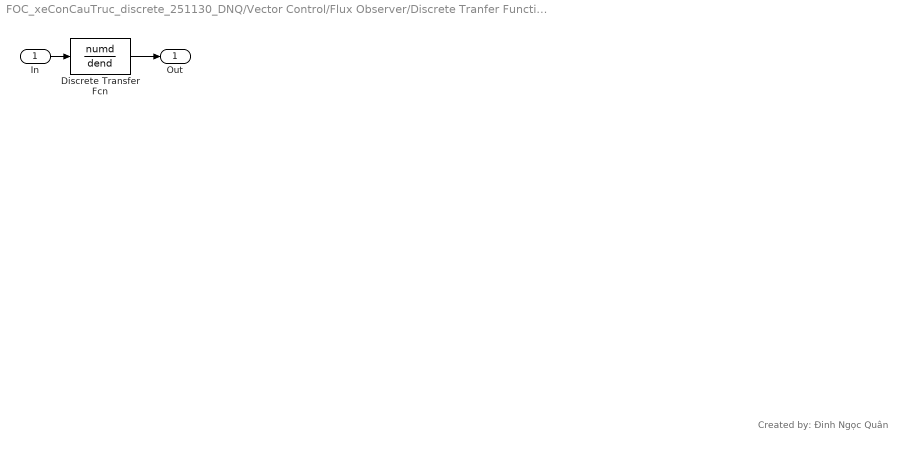
== system FOC_xeConCauTruc_discrete_251130_DNQ/Vector Control/Flux Observer/Discrete Tranfer Function1 ==
  note: Created by: Đinh Ngọc Quân
  In : Inport
  Discrete Transfer Fcn : DiscreteTransferFcn  LoadFcn=dspblkCoreblockFVToolHelper(gcbh,'load');  Numerator=numd  Denominator=dend  SampleTime=Tsample
      settings: CopyFcn=dspblkCoreblockFVToolHelper(gcbh,'copy');  DeleteFcn=dspblkCoreblockFVToolHelper(gcbh,'close');  ModelCloseFcn=dspblkCoreblockFVToolHelper(gcbh,'close');  PreSaveFcn=dspblkCoreblockFVToolHelper(gcbh,'presave');  PostSaveFcn=dspblkCoreblockFVToolHelper(gcbh,'postsave');  CloseFcn=dspblkCoreblockFVToolHelper(gcbh,'close');
  Out : Outport  InitialOutput=0  VectorParamsAs1DForOutWhenUnconnected=off
  wires:
  Discrete Transfer Fcn/1 -> Out/1
  In/1 -> Discrete Transfer Fcn/1

== matlab function FOC_xeConCauTruc_discrete_251130_DNQ/SVPWM/Delay ==
  data: T1 input; T2 input; T0 input; Tcma output; Tcmb output; Tcmc output; Sn input
function [Tcma,Tcmb,Tcmc]=D(T1,T2,T0,Sn)
T=1/2000;
Udc=530;
ton1=0.25*T0;
ton2=ton1+T1/2;
ton3=ton2+T2/2;
if Sn==1
    Tcma=ton1;Tcmb=ton2;Tcmc=ton3;
elseif Sn==2;
    Tcma=ton2;Tcmb=ton1;Tcmc=ton3;
elseif Sn==3;
    Tcma=ton3;Tcmb=ton1;Tcmc=ton2;
elseif Sn==4;
    Tcma=ton3;Tcmb=ton2;Tcmc=ton1;
elseif Sn==5;
    Tcma=ton2;Tcmb=ton3;Tcmc=ton1;
else Tcma=ton1;Tcmb=ton3;Tcmc=ton2;
end

== matlab function FOC_xeConCauTruc_discrete_251130_DNQ/T_load/MATLAB Function ==
  data: a input; TL output; t input
function TL = fcn(a,t)

M = 10000;
m = 200;
muy = 0.2;
g = 9.81;
R = 0.1/2;
k = 1.2;
i = 75;

if t < 45 
F = (M+m)*(muy*g+a);
else 
F = m*(muy*g+a);
end    
    
TL = k*F*R/i;


end

== matlab function FOC_xeConCauTruc_discrete_251130_DNQ/SVPWM/Sn ==
  data: Sn output; Ux input; Uy input
function Sn = S(Ux,Uy)
theta=atan2(Uy,Ux)*180/pi;
if theta>=0&&theta<60
    Sn=1;
elseif theta>=60&&theta<120
    Sn=2;
elseif theta>=120&&theta<180
    Sn=3;
elseif theta>=-180&&theta<-120
    Sn=4;
elseif theta>=-120&&theta<-60
    Sn=5;
else Sn=6;
end

== matlab function FOC_xeConCauTruc_discrete_251130_DNQ/SVPWM/TxTyT0 ==
  data: Ux input; Uy input; Sn input; T1 output; T2 output; T0 output
function [T1,T2,T0]=T(Ux,Uy,Sn)
Ts=1/2000;
Udc=530;

X=sqrt(3)*Ts/Udc*Uy;
Y=sqrt(3)*Ts/2/Udc*(sqrt(3)*Ux+Uy);
Z=sqrt(3)*Ts/2/Udc*(-sqrt(3)*Ux+Uy);

if Sn==1
    T1=-Z;T2=X;
elseif Sn==2;
    T1=Z;T2=Y;
elseif Sn==3;
    T1=X;T2=-Y;
elseif Sn==4;
    T1=-X;T2=Z;
elseif Sn==5;
    T1=-Y;T2=-Z;
else T1=Y;T2=-X;
end
    
if T1+T2>Ts
    a=T1;b=T2;
    T1=a*Ts/(a+b);
    T2=b*Ts/(a+b);
end

T0=Ts-T1-T2;
